simulink model "singlephase_19EE10046"  (R2021a)
settings: Solver=VariableStepAuto  StartTime=0.0  StopTime=1  RelTol=1e-3
libraries: spsMosfetLib x4, spsCurrentMeasurementLib x2, simulink x1, spsSeriesRLCBranchLib x1, spsVoltageMeasurementLib x1, spsDCVoltageSourceLib x1, spspowerguiLib x1
settings Model: Creator=HANISHA  LastModifiedBy=HANISHA

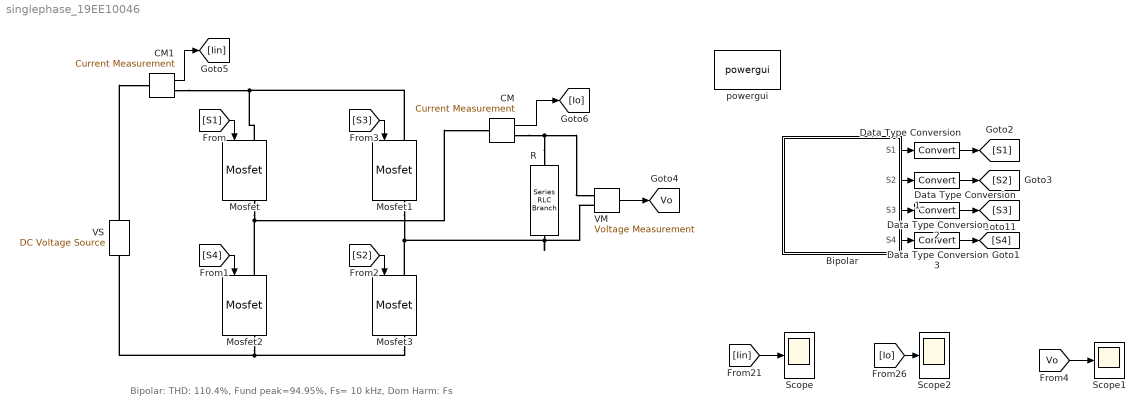
== system singlephase_19EE10046 ==
  note: Bipolar: THD: 110.4%, Fund peak=94.95%, Fs= 10 kHz, Dom Harm: Fs
  Bipolar : Subsystem
  CM : spsCurrentMeasurementLib/Current Measurement  PhasorSimulation=off  OutputType=Complex  PSBequivalent=0
  CM1 : spsCurrentMeasurementLib/Current Measurement  PhasorSimulation=off  OutputType=Complex  PSBequivalent=0
  Data Type Conversion{,1..3} (4 alike) : DataTypeConversion
  Mosfet{,1..3} (4 alike) : spsMosfetLib/Mosfet  Ron=0.02  Lon=0  Rd=0.001  Vfd=0.7  IC=0  Rs=1e5  Cs=inf  Measurements=on
  R : spsSeriesRLCBranchLib/Series RLC Branch  LConnTagsString=__new0  RConnTagsString=__new0  BranchType=R  Resistance=40  Inductance=50e-3  SetiL0=off  InitialCurrent=0  Capacitance=500e-6  Setx0=off  InitialVoltage=0  Measurements=None
  Scope : Scope
  Scope1 : Scope
  Scope2 : Scope
  VM : spsVoltageMeasurementLib/Voltage Measurement  PhasorSimulation=off  OutputType=Complex  PSBequivalent=0
  VS : spsDCVoltageSourceLib/DC Voltage Source  Amplitude=400  Measurements=None
  powergui : spspowerguiLib/powergui  Priority=1  SimulationMode=Discrete  SampleTime=1e-6  frequency=60  Iterations=50  frequencyindice=0  Pbase=100e6  ErrMax=1e-4  UnitsV=kV  UnitsW=MW  buscounter=0  FunctionMessages=off  echomessages=off  EnableUseOfTLC=off  CurrentSourceSwitches=on  DisableSnubberDevices=off  DisableRonSwitches=off  DisableVfSwitches=off  DisplayEquations=off  AutomaticDiscreteSolvers=off  SolverType=Tustin  Interpol=off  ExternalGateDelay=off  methode=off  Ts=10  x0status=blocks  SPID=off  SwTol=0  HookPort=off  NonlinearTolerance=1e-4  nMaxIteration=100  ContinueOnMaxIteration=off  RestoreLinks=warning  ResistiveCurrentMeasurement=off  Frange=[0:2:500]  Ylog=off  Xlog=on  ShowGrid=off  save=off  variable=ZData  structure=vo  ZoomFFT=off  StartTime=0.3  cycles=20  DisplayStyle=1  fundamental=50  FreqAxis=off  MaxFrequency=25000  frequencyindicesteady=1  RmsSteady=1  display=off
  tag scope: Vo=global
  wires:
  CM/1 -> [Io]
  [S1] -> Mosfet/1
  [S3] -> Mosfet1/1
  CM1/1 -> [Iin]
  [S2] -> Mosfet3/1
  [S4] -> Mosfet2/1
  VM/1 -> [Vo]
  Bipolar/4(S4) -> Data Type Conversion3/1
  Bipolar/1(S1) -> Data Type Conversion/1
  Data Type Conversion2/1 -> [S3]
  Data Type Conversion/1 -> [S1]
  Bipolar/2(S2) -> Data Type Conversion1/1
  Bipolar/3(S3) -> Data Type Conversion2/1
  Data Type Conversion3/1 -> [S4]
  Data Type Conversion1/1 -> [S2]
  [Iin] -> Scope/1
  [Io] -> Scope2/1
  [Vo] -> Scope1/1
  connections:
  Mosfet/LConn1 -- CM1/RConn1 -- Mosfet1/LConn1
  R/LConn1 -- CM/RConn1 -- VM/LConn1
  Mosfet2/RConn1 -- VS/LConn1 -- Mosfet3/RConn1
  Mosfet/RConn1 -- CM/LConn1 -- Mosfet2/LConn1
  R/RConn1 -- Mosfet3/LConn1 -- Mosfet1/RConn1 -- VM/LConn2
  VS/RConn1 -- CM1/LConn1

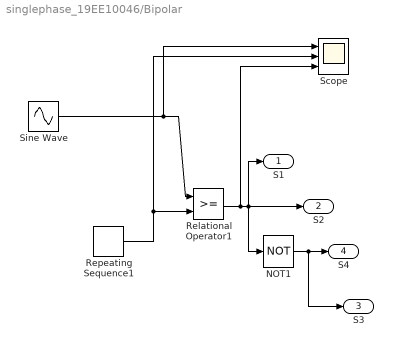
== system singlephase_19EE10046/Bipolar ==
  NOT1 : Logic  Operator=NOT  AllPortsSameDT=off  OutDataTypeStr=boolean
  Relational Operator1 : RelationalOperator  OutDataTypeStr=boolean  RndMeth=Nearest
  Repeating Sequence1 : simulink/Sources/Repeating Sequence  rep_seq_t=[0 0.00001 0.00002 0.00003 0.00004]  rep_seq_y=[0 1 0 -1 0]
  Scope : Scope  NumInputPorts=3
  Sine Wave : Sin  Amplitude=.95  Frequency=2*pi*50  SampleTime=0
  S1 : Outport
  S2 : Outport  Port=2
  S3 : Outport  Port=3
  S4 : Outport  Port=4
  wires:
  Sine Wave/1 -> Scope/1, Relational Operator1/1
  Relational Operator1/1 -> Scope/3, S1/1, S2/1, NOT1/1
  NOT1/1 -> S3/1, S4/1
  Repeating Sequence1/1 -> Scope/2, Relational Operator1/2
